simulink model "Lab02"  (Simulink 7.4)
settings: Solver=ode45  StartTime=0.0  StopTime=10  RelTol=1e-3
libraries: cstblocks x5, dspsrcs4 x1
settings Model: Creator=AshfaqAhmad  LastModifiedBy=AshfaqAhmad

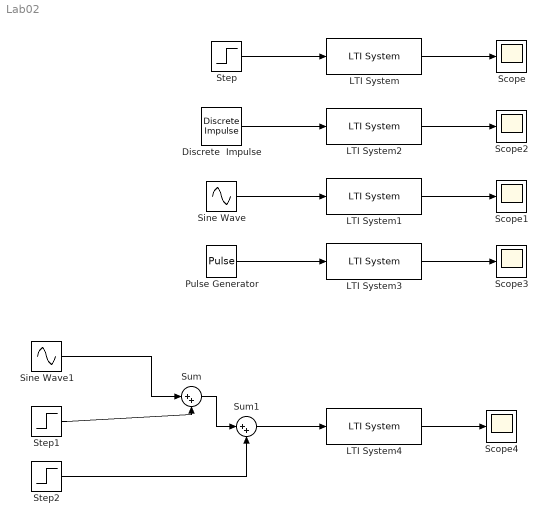
== system Lab02 ==
  Discrete  Impulse : dspsrcs4/Discrete  Impulse  Delay=0  SampleTime=1  FrameSample=1  dataType=double  isSigned=on  wordLen=16  udDataType=sfix(16)  fracBitsMode=Best precision  numFracBits=15
  LTI System{,1..4} (5 alike) : cstblocks/LTI System  SystemSampleTime=-1  sys=tf(100,[1 4 20])  IC=[]
  Pulse Generator : DiscretePulseGenerator  PulseType=Time based  Amplitude=2  Period=10  PulseWidth=5  PhaseDelay=0  SampleTime=1
  Scope{,1..4} (5 alike) : Scope
      Scope2 settings: SaveName=ScopeData2
      Scope3 settings: SaveName=ScopeData3
      Scope4 settings: SaveName=ScopeData4
  Sine Wave : Sin  Amplitude=1  Bias=0  Frequency=1  Phase=0  Samples=10  SampleTime=0  Offset=0
  Sine Wave1 : Sin  TimeSource=Use external signal  Amplitude=1  Bias=0  Frequency=2  Phase=0  Samples=10  SampleTime=0  Offset=0
  Step : Step  SampleTime=0
  Step1 : Step  SampleTime=0.01
  Step2 : Step  Time=5  SampleTime=0.01
  Sum : Sum  Inputs=|++  OutDataType=fixdt(1, 16)  OutScaling=2^0
  Sum1 : Sum  Inputs=|++  OutDataType=fixdt(1, 16)  OutScaling=2^0
  wires:
  Step/1 -> LTI System/1
  LTI System/1 -> Scope/1
  Sine Wave/1 -> LTI System1/1
  LTI System1/1 -> Scope1/1
  Discrete  Impulse/1 -> LTI System2/1
  LTI System2/1 -> Scope2/1
  Pulse Generator/1 -> LTI System3/1
  Step1/1 -> Sum/2
  Sine Wave1/1 -> Sum/1
  Step2/1 -> Sum1/2
  Sum/1 -> Sum1/1
  Sum1/1 -> LTI System4/1
  LTI System4/1 -> Scope4/1
  LTI System3/1 -> Scope3/1
